simulink model "model_test"  (R2023a)
settings: Solver=VariableStepAuto  StartTime=0.0  StopTime=10.0  RelTol=1e-3
values from neighbouring files (symbols this model uses):
  a = 1    [script_test.m]
  b = 2    [script_test.m]
  c = 3    [script_test.m]
settings Model: Creator=AdrianNegoita  LastModifiedBy=AdrianNegoita

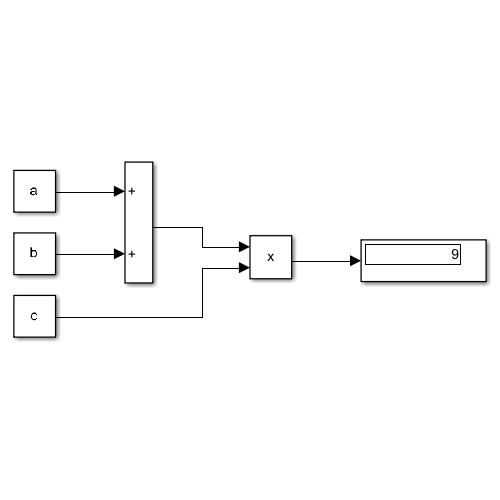
[thumbnail: Simulink's stored preview of the top-level diagram]
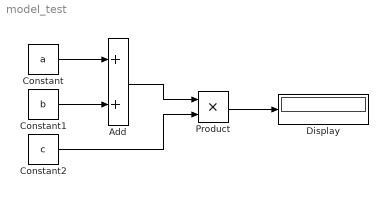
== system model_test ==
  Add : Sum
  Constant : Constant  Value=a
  Constant1 : Constant  Value=b
  Constant2 : Constant  Value=c
  Display : Display
  Product : Product
  wires:
  Constant/1 -> Add/1
  Constant1/1 -> Add/2
  Constant2/1 -> Product/2
  Add/1 -> Product/1
  Product/1 -> Display/1
